simulink model "fixpt_dt_disp"  (R2015b)
settings: Solver=ode45  SolverMode=SingleTasking  StartTime=0.0  StopTime=10.0  RelTol=1e-3
settings Model: Creator=amatsumo  LastModifiedBy=amatsumo
settings DataIOCC: SaveFormat=Array  SaveOutput=off  SignalLogging=off  SaveTime=off
settings OptimizationCC: BlockReduction=off  ConditionallyExecuteInputs=off  DefaultParameterBehavior=Inlined
settings DebuggingCC: AlgebraicLoopMsg=error  UnderspecifiedInitializationDetection=Classic  MergeDetectMultiDrivingBlocksExec=none  SolverPrmCheckMsg=warning  InheritedTsInSrcMsg=none  SingleTaskRateTransMsg=error  StateNameClashWarn=warning
settings HardwareCC: ProdBitPerPointer=32  ProdLargestAtomicFloat=None  ProdIntDivRoundTo=Undefined  ProdEndianess=Unspecified  ProdWordSize=32  ProdHWDeviceType=ASIC/FPGA->ASIC/FPGA  ProdEqTarget=off
settings GRTTargetCC: GeneratePreprocessorConditionals=Disable all
settings ConfigComp: CovModelRefEnable=Off  CovSFcnEnable=off

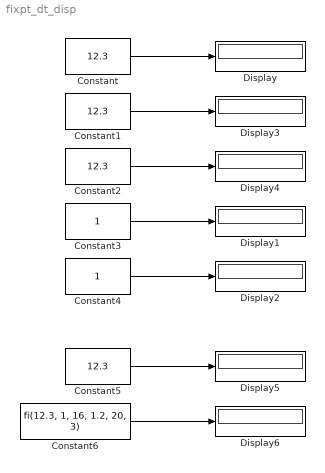
== system fixpt_dt_disp ==
  Constant : Constant  Value=12.3  OutDataTypeStr=fixdt(1,16,4)  SampleTime=1
  Constant1 : Constant  Value=12.3  OutDataTypeStr=fixdt(0,16,4)  SampleTime=1
  Constant2 : Constant  Value=12.3  OutDataTypeStr=fixdt(0,16,-4)  SampleTime=1
  Constant3 : Constant  OutDataTypeStr=boolean  SampleTime=1
  Constant4 : Constant  OutDataTypeStr=fixdt(0,1,0)  SampleTime=1
  Constant5 : Constant  Value=12.3  OutDataTypeStr=fixdt(1,16,1.2,1)  SampleTime=1
  Constant6 : Constant  Value=fi(12.3, 1, 16, 1.2, 20, 3)  SampleTime=1
  Display{,1..6} (7 alike) : Display
  wires:
  Constant/1 -> Display/1
  Constant1/1 -> Display3/1
  Constant2/1 -> Display4/1
  Constant3/1 -> Display1/1
  Constant4/1 -> Display2/1
  Constant5/1 -> Display5/1
  Constant6/1 -> Display6/1
